simulink model "matlab_converter"  (R2016a)
settings: Solver=VariableStepAuto  StartTime=0.0  StopTime=5  RelTol=1e-3
libraries: powerlib x11, powerlib_meascontrol x1
settings Model: Creator=Vaishusegarr  LastModifiedBy=Vaishusegarr

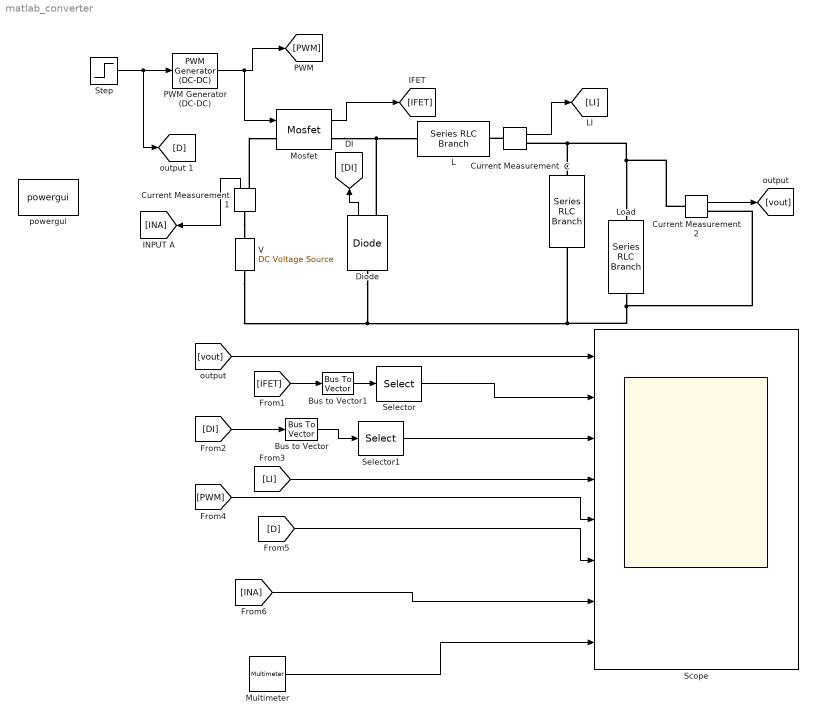
== system matlab_converter ==
  " Load " : powerlib/Elements/Series RLC Branch  LConnTagsString=__new0  RConnTagsString=__new0  BranchType=R  Resistance=2.4  Inductance=1e-3  SetiL0=off  InitialCurrent=0  Capacitance=1e-6  Setx0=off  InitialVoltage=0  Measurements=Branch voltage and current
  " C " : powerlib/Elements/Series RLC Branch  LConnTagsString=__new0  RConnTagsString=__new0  BranchType=C  Resistance=1  Inductance=1e-3  SetiL0=off  InitialCurrent=0  Capacitance=15.625e-6  Setx0=off  InitialVoltage=0  Measurements=Branch voltage and current
  Bus to Vector : BusToVector
  Bus to Vector1 : BusToVector
  Current Measurement : powerlib/Measurements/Current Measurement  PhasorSimulation=off  OutputType=Complex  PSBequivalent=0
  Current Measurement1 : powerlib/Measurements/Current Measurement  PhasorSimulation=off  OutputType=Complex  PSBequivalent=0
  Current Measurement2 : powerlib/Measurements/Current Measurement  PhasorSimulation=off  OutputType=Complex  PSBequivalent=0
  Diode : powerlib/Power Electronics/Diode  Ron=1e-3  Lon=0  Vf=0  IC=0  UseSnubber=off  Rs=inf  Cs=inf  Measurements=on
  "L " : powerlib/Elements/Series RLC Branch  LConnTagsString=__new0  RConnTagsString=__new0  BranchType=L  Resistance=1  Inductance=0.3e-3  SetiL0=off  InitialCurrent=0  Capacitance=1e-6  Setx0=off  InitialVoltage=0  Measurements=Branch voltage and current
  Mosfet : powerlib/Power Electronics/Mosfet  Ron=1e-3  Lon=0  Rd=1e-3  Vfd=0  IC=0  Rs=inf  Cs=inf  Measurements=on
  Multimeter : powerlib/Measurements/Multimeter  PhasorSimulation=off  OutputType=Complex  sel=4  L=7  Gain=1  yselected={'Usrc: V '};  PSBOutputType=1  PSBequivalent=0  AxesSetting=[0,0.1,-100,100]  Display=0  SavedBlockNames=-11
  PWM Generator (DC-DC) : powerlib_meascontrol/Pulse & Signal Generators/PWM Generator (DC-DC)  Fsw=20000  Ts=0
  Scope : Scope  NumInputPorts=8
  Selector : Selector  InputPortWidth=2  IndexOptions=Index vector (dialog)  Indices=1  OutputSizes=1
  Selector1 : Selector  InputPortWidth=2  IndexOptions=Index vector (dialog)  Indices=1  OutputSizes=1
  Step : Step  Time=0.015  Before=0.25  After=0.25  SampleTime=0
  "V " : powerlib/Electrical Sources/DC Voltage Source  Amplitude=48  Measurements=Voltage
  powergui : powerlib/powergui  Priority=1  SimulationMode=Continuous  SolverType=Tustin/Backward Euler (TBE)  SampleTime=50e-6  frequency=60  SPID=on  DisableSnubberDevices=on  DisableRonSwitches=off  DisableVfSwitches=off  SwTol=0  DisplayEquations=off  Interpol=off  ExternalGateDelay=off  methode=off  Ts=10  FunctionMessages=off  echomessages=off  HookPort=off  EnableUseOfTLC=off  x0status=blocks  frequencyindice=0  Pbase=100e6  ErrMax=1e-4  Iterations=50  UnitsV=kV  UnitsW=MW  buscounter=0  RestoreLinks=warning  ResistiveCurrentMeasurement=off  Frange=[0:2:500]  Ylog=off  Xlog=on  ShowGrid=off  save=off  variable=ZData  structure=0  ZoomFFT=off  StartTime=0.0  cycles=1  DisplayStyle=1  fundamental=60  FreqAxis=off  MaxFrequency=1000  frequencyindicesteady=1  RmsSteady=1  display=off
  wires:
  Step/1 -> [D], PWM Generator (DC-DC)/1
  Current Measurement/1 -> [LI]
  Diode/1 -> [DI]
  Mosfet/1 -> [IFET]
  PWM Generator (DC-DC)/1 -> Mosfet/1, [PWM]
  [LI] -> Scope/4
  [D] -> Scope/6
  [PWM] -> Scope/5
  [vout] -> Scope/1
  [DI] -> Bus to Vector/1
  [IFET] -> Bus to Vector1/1
  Bus to Vector1/1 -> Selector/1
  Selector/1 -> Scope/2
  Bus to Vector/1 -> Selector1/1
  Selector1/1 -> Scope/3
  Current Measurement1/1 -> [INA]
  [INA] -> Scope/7
  Multimeter/1 -> Scope/8
  Current Measurement2/1 -> [vout]
  connections:
  Mosfet/RConn1 -- Diode/RConn1 -- "L "/LConn1
  Current Measurement/LConn1 -- "L "/RConn1
  " C "/LConn1 -- Current Measurement2/LConn1 -- " Load "/LConn1 -- Current Measurement/RConn1
  Current Measurement1/LConn1 -- "V "/RConn1
  Current Measurement1/RConn1 -- Mosfet/LConn1
  "V "/LConn1 -- Diode/LConn1 -- " Load "/RConn1 -- Current Measurement2/RConn1 -- " C "/RConn1
